simulink library "Library_SII_2018"  (R2018b)
settings: Solver=ode45  StartTime=0.0  StopTime=10.0  RelTol=1e-3  EnableMultiTasking=on
undefined symbols (not defined in the file or in its folder): coder, gcbh, r, simscape
libraries: fl_lib x157, nesl_utility x81, Library_SII2 x44, simulink x17, powerlib x12, mblibv1 x11, Simscape_SII_lib x11, elec_lib x10, Pneumatic_lib x4, $bdroot x2, peRmsMeasurement x1, powerlib_extras x1
(part 5 of 6)

== system Library_SII_2018/Mécanique/Engrenage droit SS ==
  Capteur de puissance mécanique de rotation : Subsystem  mask(Capteur de puissance mécanique de rotation){}
      mask help:
      | Le bloc représente un capteur de puissance mécanique de rotation.
      | R et C sont des ports physiques conservatifs.
      |
      | P, T et W sont des ports Simulink délivrant les valeurs de :
      |  - la puissance mécanique traversant le bloc (en W)
      |  - le couple transmis à travers le bloc (en Nm)
      |  - la vitesse de rotation (en rad/s)
      |
      | Ces valeurs sont calculées par rapport au référentiel Ref.
      mask Display:
      | plot([149.600878633536;150.016472378793;150.47508104106;150.972287968219;151.50330478576;152.063017511447;152.646035805762;153.246744883819;153.859359588817;154.477980106257;155.096648782383;155.709407499646;156.310355056631;156.893703999851;157.453836360095;157.985357756531;158.483149347555;158.942417128023;159.358738098149;159.728102859405;160.046954227227;160.312221488639;160.521349974904;160.672325664379;160.763694578642;160.794576785101;160.764674871227;160.674276808796;160.524253180566;160.316048796087;160.051668777399;159.733659248606;159.365082815313;158.949489070056;158.490880407788;157.993673480629;157.462656663088;156.908284800231], [156.971389291536;157.430657072004;157.84697804213;158.216342803387;158.535194171208;158.80046143262;159.009589918885;159.16056560836;159.251934522623;159.282816729083;159.252914815208;159.162516752777;159.012493124547;158.804288740068;158.53990872138;158.221899192587;157.853322759294;157.437729014037;156.979120351769;156.48191342461;155.950896607069;155.391183881382;154.808165587067;154.20745650901;153.594841804012;152.976221286573;152.357552610446;151.744793893183;151.143846336199;150.560497392978;150.000365032735;149.468843636298;148.971052045274;148.511784264806;148.095463294681;147.726098533424;147.407247165603;147.144199990631])
      | plot([152.057635404444;152.93604260309;153.834625296826;154.744729643097;155.657590839533;156.564417533794;157.45647648909;158.325176690034;159.162152078811;159.959342124889;160.709069452336;161.404113777147;162.037781442523;162.603969882449;163.097226392739;163.512800643557;163.846690427691;164.095680203997;164.257372064819;164.330208829146;164.313489039122;164.27939575172], [142.228020686971;141.979030910664;141.817339049842;141.744502285515;141.761222075539;141.867337399197;142.061826307913;142.342815767178;142.707599694895;143.152665022428;143.673725527376;144.265763112236;144.923076131425;145.639334301243;146.40763966397;147.220593018964;148.070365181011;148.948772379657;149.847355073393;150.757459419663;151.6703206161;152.055850472277])
      | %plot([116.468514315784;116.438789536125;116.349901463023;116.202706137216;115.998621130155;115.739611892022;115.42817282337;115.067303252679;114.660478551187;114.211616663162;113.725040373958;113.205435679231;112.657806656235;112.087427271827;111.499790591278;110.900555877058;110.29549408704;109.690432297022;109.091197582803;108.503560902254;107.933181517846;107.38555249485;106.865947800123;106.379371510919;105.930509622894;105.523684921402;105.162815350711;104.851376282059;104.592367043926;104.388282036865;104.241086711057;104.152198637956;104.122473858297;104.152198637956;104.241086711057;104.388282036865;104.592367043926;104.851376282059;105.162815350711;105.523684921402;105.930509622894;106.379371510919;106.865947800123;107.38555249485;107.933181517846;108.503560902254;109.091197582803;109.690432297022;110.29549408704;110.900555877058;111.499790591278;112.087427271827;112.657806656235;113.205435679231;113.725040373958;114.211616663162;114.660478551187;115.067303252679;115.42817282337;115.739611892022;115.998621130155;116.202706137216;116.349901463023;116.438789536125;116.468514315784;116.468514315784], [111.618284136057;111.013222346039;110.413987631819;109.826350951271;109.255971566862;108.708342543866;108.188737849139;107.702161559936;107.253299671911;106.846474970419;106.485605399728;106.174166331075;105.915157092943;105.711072085881;105.563876760074;105.474988686973;105.445263907313;105.474988686973;105.563876760074;105.711072085881;105.915157092943;106.174166331075;106.485605399728;106.846474970419;107.253299671911;107.702161559936;108.188737849139;108.708342543866;109.255971566862;109.826350951271;110.413987631819;111.013222346039;111.618284136057;112.223345926075;112.822580640295;113.410217320843;113.980596705252;114.528225728247;115.047830422975;115.534406712178;115.983268600203;116.390093301695;116.750962872386;117.062401941038;117.321411179171;117.525496186232;117.67269151204;117.761579585141;117.7913043648;117.761579585141;117.67269151204;117.525496186232;117.321411179171;117.062401941038;116.750962872386;116.390093301695;115.983268600203;115.534406712178;115.047830422975;114.528225728247;113.980596705252;113.410217320843;112.822580640295;112.223345926075;111.618284136057;111.618284136057])
      | plot([239.23602886498;238.828071429858;237.608127977604;235.587947230552;232.78698463364;229.232214987837;224.957872668068;220.005121927465;214.421660463109;208.261260061133;201.583248745024;194.451939414329;186.936010476274;179.107844435155;171.042830809261;162.818640088593;154.514475725591;146.210311362589;137.986120641921;129.921107016027;122.092940974909;114.577012036853;107.445702706158;100.76769139005;94.607290988073;89.0238295237172;84.0710787831142;79.7967364633452;76.2419668175427;73.4410042206305;71.4208234735788;70.2008800213248;69.7929225862026;70.2008800213248;71.4208234735788;73.4410042206306;76.2419668175428;79.7967364633454;84.0710787831144;89.0238295237174;94.6072909880733;100.76769139005;107.445702706159;114.577012036853;122.092940974909;129.921107016027;137.986120641921;146.210311362589;154.514475725591;162.818640088593;171.042830809261;179.107844435155;186.936010476274;194.451939414329;201.583248745024;208.261260061133;214.421660463109;220.005121927465;224.957872668068;229.232214987837;232.78698463364;235.587947230552;237.608127977604;238.828071429858;239.23602886498;239.23602886498], [155.774275772274;147.47628550917;139.258209428443;131.199192095207;123.376846251889;115.866505365088;108.740498123116;102.067451871182;95.9116316925529;90.3323215006612;85.3832531026163;81.1120887325275;77.5599620381344;74.7610819412943;72.742403187363;71.5233667562631;71.1157126352191;71.5233667562631;72.742403187363;74.7610819412943;77.5599620381345;81.1120887325275;85.3832531026164;90.3323215006612;95.9116316925529;102.067451871182;108.740498123116;115.866505365089;123.376846251889;131.199192095207;139.258209428443;147.47628550917;155.774275772274;164.072266035377;172.290342116104;180.34935944934;188.171705292658;195.682046179459;202.808053421432;209.481099673365;215.636919851994;221.216230043886;226.165298441931;230.43646281202;233.988589506413;236.787469603253;238.806148357184;240.025184788284;240.432838909328;240.025184788284;238.806148357184;236.787469603253;233.988589506413;230.43646281202;226.165298441931;221.216230043886;215.636919851994;209.481099673365;202.808053421432;195.682046179459;188.171705292658;180.34935944934;172.290342116105;164.072266035378;155.774275772274;155.774275772274])
      | plot([252.715889364481;252.243022716633;250.828976737403;248.487369462568;245.240751850236;241.120390602797;236.165967051481;230.425195003451;223.953361231755;216.812793033479;209.072257983804;200.806301666664;192.094529760025;183.020841389688;173.672621134841;164.139897466795;154.514475725591;144.889053984387;135.356330316341;126.008110061494;116.934421691157;108.222649784518;99.9566934673787;92.2161584177032;85.075590219427;78.6037564477313;72.8629843997015;67.9085608483856;63.7881996009461;60.5415819886144;58.199974713779;56.7859287345493;56.3130620867014;56.7859287345493;58.1999747137791;60.5415819886146;63.7881996009463;67.9085608483858;72.8629843997018;78.6037564477315;85.0755902194273;92.2161584177035;99.9566934673791;108.222649784519;116.934421691157;126.008110061494;135.356330316341;144.889053984387;154.514475725591;164.139897466796;173.672621134841;183.020841389688;192.094529760025;200.806301666664;209.072257983803;216.812793033479;223.953361231755;230.425195003451;236.165967051481;241.120390602797;245.240751850236;248.487369462568;250.828976737403;252.243022716633;252.715889364481;252.715889364481], [154.514475725591;144.895228084285;135.36861905618;126.026395093992;116.958526921455;108.252343066071;99.9916888376535;92.2561188521535;85.1201308772245;78.6524483779929;72.9153586725213;67.9641130708855;63.8463947748555;60.6018596625959;58.2617543808809;56.8486154228053;56.3760520890355;56.8486154228053;58.2617543808809;60.6018596625959;63.8463947748555;67.9641130708856;72.9153586725213;78.652448377993;85.1201308772246;92.2561188521536;99.9916888376536;108.252343066072;116.958526921455;126.026395093992;135.36861905618;144.895228084285;154.514475725591;164.133723366898;173.660332395002;183.002556357191;192.070424529728;200.776608385111;209.037262613529;216.772832599029;223.908820573958;230.37650307319;236.113592778661;241.064838380297;245.182556676327;248.427091788587;250.767197070302;252.180336028377;252.652899362147;252.180336028377;250.767197070301;248.427091788587;245.182556676327;241.064838380297;236.113592778661;230.37650307319;223.908820573958;216.772832599029;209.037262613529;200.776608385111;192.070424529728;183.002556357191;173.660332395002;164.133723366898;154.514475725592;154.514475725591])
      | plot([154.514475725591;129.948374815285;179.017586633563;154.514475725591], [240.369848906994;203.583687543869;203.583687543869;240.369848906994])
      | %plot([105.382273904979;149.60125554353], [115.271704271436;156.971085816622])
      | plot([144.688035361469;144.688035361469], [152.057865634561;203.583687543869])
      | plot([164.277926087379;164.277926087379], [152.057865634561;203.583687543869])
      | plot([159.112745895982;159.616665914655], [149.60125554353;149.60125554353])
      | %plot([115.208714269102;159.364705905318], [107.901873998344;149.60125554353])
      | plot([0;311.800511553884;311.800511553884;0;0], [311.800511553884;311.800511553884;0;0;311.800511553884])
      | ;
      | color('red');
      | port_label('LConn', 1,'R')
      | port_label('RConn', 1,'C')
      | port_label('LConn', 2,'Ref')
      | port_label('output', 1,'P')
      | port_label('output', 2,'T')
      | port_label('output', 3,'W')
      | %port_label('RConn', 3,'A')
  Couple d'entrée : Scope
  Couple de sortie : Scope
  Gain : Gain  Gain=1-n
  Gear Box : fl_lib/Mechanical/Mechanisms/Gear Box  ratio=r  t_in_specify=off  t_in_priority=High  t_in=0 N*m  t_in_nominal_specify=off  t_in_nominal_unit=N*m  t_in_nominal_value=1  t_out_specify=off  t_out_priority=High  t_out=0 N*m  t_out_nominal_specify=off  t_out_nominal_unit=N*m  t_out_nominal_value=1
  Ideal Torque Source : fl_lib/Mechanical/Mechanical Sources/Ideal Torque Source
  Inertia : fl_lib/Mechanical/Rotational Elements/Inertia  inertia=J kg*m^2  w_specify=on  w_priority=High  w=0 rad/s  w_nominal_specify=off  w_nominal_unit=rad/s  w_nominal_value=1  t_specify=off  t_priority=High  t=0 N*m  t_nominal_specify=off  t_nominal_unit=N*m  t_nominal_value=1
  Simulink-PS Converter : nesl_utility/Simulink-PS Converter  PhysicalDomain=network_engine_domain  SubClassName=ps_input  LeftPortType=input  RightPortType=output  PseudoPeriodic=off  Frequencies=[]  NoiseDistribution=none  NoiseParameters=[]  Unit=1  AffineConversion=off  FilteringAndDerivatives=zero  SimscapeFilterOrder=1  InputFilterTimeConstant=.001  UdotUserProvided=0
  R : PMIOPort  Side=Right
  V : PMIOPort  Tag=PMCPort  Port=2  Side=Left
  Ref : PMIOPort  Tag=PMCPort  Port=3  Side=Left
  wires:
  Capteur de puissance mécanique de rotation/2(C) -> Gain/1, Couple d'entrée/1
  Gain/1 -> Simulink-PS Converter/1, Couple de sortie/1
  connections:
  V/RConn1 -- Capteur de puissance mécanique de rotation/LConn2
  Capteur de puissance mécanique de rotation/LConn1 -- Ideal Torque Source/RConn2 -- Ref/RConn1
  R/RConn1 -- Gear Box/RConn1
  Simulink-PS Converter/RConn1 -- Ideal Torque Source/RConn1
  Inertia/LConn1 -- Gear Box/LConn1 -- Ideal Torque Source/LConn1 -- Capteur de puissance mécanique de rotation/RConn1

== system Library_SII_2018/Mécanique/Roue - Vis sans fin SS ==
  Capteur de puissance mécanique de rotation : Subsystem  mask(Capteur de puissance mécanique de rotation){}
      mask help:
      | Le bloc représente un capteur de puissance mécanique de rotation.
      | R et C sont des ports physiques conservatifs.
      |
      | P, T et W sont des ports Simulink délivrant les valeurs de :
      |  - la puissance mécanique traversant le bloc (en W)
      |  - le couple transmis à travers le bloc (en Nm)
      |  - la vitesse de rotation (en rad/s)
      |
      | Ces valeurs sont calculées par rapport au référentiel Ref.
      mask Display:
      | plot([149.600878633536;150.016472378793;150.47508104106;150.972287968219;151.50330478576;152.063017511447;152.646035805762;153.246744883819;153.859359588817;154.477980106257;155.096648782383;155.709407499646;156.310355056631;156.893703999851;157.453836360095;157.985357756531;158.483149347555;158.942417128023;159.358738098149;159.728102859405;160.046954227227;160.312221488639;160.521349974904;160.672325664379;160.763694578642;160.794576785101;160.764674871227;160.674276808796;160.524253180566;160.316048796087;160.051668777399;159.733659248606;159.365082815313;158.949489070056;158.490880407788;157.993673480629;157.462656663088;156.908284800231], [156.971389291536;157.430657072004;157.84697804213;158.216342803387;158.535194171208;158.80046143262;159.009589918885;159.16056560836;159.251934522623;159.282816729083;159.252914815208;159.162516752777;159.012493124547;158.804288740068;158.53990872138;158.221899192587;157.853322759294;157.437729014037;156.979120351769;156.48191342461;155.950896607069;155.391183881382;154.808165587067;154.20745650901;153.594841804012;152.976221286573;152.357552610446;151.744793893183;151.143846336199;150.560497392978;150.000365032735;149.468843636298;148.971052045274;148.511784264806;148.095463294681;147.726098533424;147.407247165603;147.144199990631])
      | plot([152.057635404444;152.93604260309;153.834625296826;154.744729643097;155.657590839533;156.564417533794;157.45647648909;158.325176690034;159.162152078811;159.959342124889;160.709069452336;161.404113777147;162.037781442523;162.603969882449;163.097226392739;163.512800643557;163.846690427691;164.095680203997;164.257372064819;164.330208829146;164.313489039122;164.27939575172], [142.228020686971;141.979030910664;141.817339049842;141.744502285515;141.761222075539;141.867337399197;142.061826307913;142.342815767178;142.707599694895;143.152665022428;143.673725527376;144.265763112236;144.923076131425;145.639334301243;146.40763966397;147.220593018964;148.070365181011;148.948772379657;149.847355073393;150.757459419663;151.6703206161;152.055850472277])
      | %plot([116.468514315784;116.438789536125;116.349901463023;116.202706137216;115.998621130155;115.739611892022;115.42817282337;115.067303252679;114.660478551187;114.211616663162;113.725040373958;113.205435679231;112.657806656235;112.087427271827;111.499790591278;110.900555877058;110.29549408704;109.690432297022;109.091197582803;108.503560902254;107.933181517846;107.38555249485;106.865947800123;106.379371510919;105.930509622894;105.523684921402;105.162815350711;104.851376282059;104.592367043926;104.388282036865;104.241086711057;104.152198637956;104.122473858297;104.152198637956;104.241086711057;104.388282036865;104.592367043926;104.851376282059;105.162815350711;105.523684921402;105.930509622894;106.379371510919;106.865947800123;107.38555249485;107.933181517846;108.503560902254;109.091197582803;109.690432297022;110.29549408704;110.900555877058;111.499790591278;112.087427271827;112.657806656235;113.205435679231;113.725040373958;114.211616663162;114.660478551187;115.067303252679;115.42817282337;115.739611892022;115.998621130155;116.202706137216;116.349901463023;116.438789536125;116.468514315784;116.468514315784], [111.618284136057;111.013222346039;110.413987631819;109.826350951271;109.255971566862;108.708342543866;108.188737849139;107.702161559936;107.253299671911;106.846474970419;106.485605399728;106.174166331075;105.915157092943;105.711072085881;105.563876760074;105.474988686973;105.445263907313;105.474988686973;105.563876760074;105.711072085881;105.915157092943;106.174166331075;106.485605399728;106.846474970419;107.253299671911;107.702161559936;108.188737849139;108.708342543866;109.255971566862;109.826350951271;110.413987631819;111.013222346039;111.618284136057;112.223345926075;112.822580640295;113.410217320843;113.980596705252;114.528225728247;115.047830422975;115.534406712178;115.983268600203;116.390093301695;116.750962872386;117.062401941038;117.321411179171;117.525496186232;117.67269151204;117.761579585141;117.7913043648;117.761579585141;117.67269151204;117.525496186232;117.321411179171;117.062401941038;116.750962872386;116.390093301695;115.983268600203;115.534406712178;115.047830422975;114.528225728247;113.980596705252;113.410217320843;112.822580640295;112.223345926075;111.618284136057;111.618284136057])
      | plot([239.23602886498;238.828071429858;237.608127977604;235.587947230552;232.78698463364;229.232214987837;224.957872668068;220.005121927465;214.421660463109;208.261260061133;201.583248745024;194.451939414329;186.936010476274;179.107844435155;171.042830809261;162.818640088593;154.514475725591;146.210311362589;137.986120641921;129.921107016027;122.092940974909;114.577012036853;107.445702706158;100.76769139005;94.607290988073;89.0238295237172;84.0710787831142;79.7967364633452;76.2419668175427;73.4410042206305;71.4208234735788;70.2008800213248;69.7929225862026;70.2008800213248;71.4208234735788;73.4410042206306;76.2419668175428;79.7967364633454;84.0710787831144;89.0238295237174;94.6072909880733;100.76769139005;107.445702706159;114.577012036853;122.092940974909;129.921107016027;137.986120641921;146.210311362589;154.514475725591;162.818640088593;171.042830809261;179.107844435155;186.936010476274;194.451939414329;201.583248745024;208.261260061133;214.421660463109;220.005121927465;224.957872668068;229.232214987837;232.78698463364;235.587947230552;237.608127977604;238.828071429858;239.23602886498;239.23602886498], [155.774275772274;147.47628550917;139.258209428443;131.199192095207;123.376846251889;115.866505365088;108.740498123116;102.067451871182;95.9116316925529;90.3323215006612;85.3832531026163;81.1120887325275;77.5599620381344;74.7610819412943;72.742403187363;71.5233667562631;71.1157126352191;71.5233667562631;72.742403187363;74.7610819412943;77.5599620381345;81.1120887325275;85.3832531026164;90.3323215006612;95.9116316925529;102.067451871182;108.740498123116;115.866505365089;123.376846251889;131.199192095207;139.258209428443;147.47628550917;155.774275772274;164.072266035377;172.290342116104;180.34935944934;188.171705292658;195.682046179459;202.808053421432;209.481099673365;215.636919851994;221.216230043886;226.165298441931;230.43646281202;233.988589506413;236.787469603253;238.806148357184;240.025184788284;240.432838909328;240.025184788284;238.806148357184;236.787469603253;233.988589506413;230.43646281202;226.165298441931;221.216230043886;215.636919851994;209.481099673365;202.808053421432;195.682046179459;188.171705292658;180.34935944934;172.290342116105;164.072266035378;155.774275772274;155.774275772274])
      | plot([252.715889364481;252.243022716633;250.828976737403;248.487369462568;245.240751850236;241.120390602797;236.165967051481;230.425195003451;223.953361231755;216.812793033479;209.072257983804;200.806301666664;192.094529760025;183.020841389688;173.672621134841;164.139897466795;154.514475725591;144.889053984387;135.356330316341;126.008110061494;116.934421691157;108.222649784518;99.9566934673787;92.2161584177032;85.075590219427;78.6037564477313;72.8629843997015;67.9085608483856;63.7881996009461;60.5415819886144;58.199974713779;56.7859287345493;56.3130620867014;56.7859287345493;58.1999747137791;60.5415819886146;63.7881996009463;67.9085608483858;72.8629843997018;78.6037564477315;85.0755902194273;92.2161584177035;99.9566934673791;108.222649784519;116.934421691157;126.008110061494;135.356330316341;144.889053984387;154.514475725591;164.139897466796;173.672621134841;183.020841389688;192.094529760025;200.806301666664;209.072257983803;216.812793033479;223.953361231755;230.425195003451;236.165967051481;241.120390602797;245.240751850236;248.487369462568;250.828976737403;252.243022716633;252.715889364481;252.715889364481], [154.514475725591;144.895228084285;135.36861905618;126.026395093992;116.958526921455;108.252343066071;99.9916888376535;92.2561188521535;85.1201308772245;78.6524483779929;72.9153586725213;67.9641130708855;63.8463947748555;60.6018596625959;58.2617543808809;56.8486154228053;56.3760520890355;56.8486154228053;58.2617543808809;60.6018596625959;63.8463947748555;67.9641130708856;72.9153586725213;78.652448377993;85.1201308772246;92.2561188521536;99.9916888376536;108.252343066072;116.958526921455;126.026395093992;135.36861905618;144.895228084285;154.514475725591;164.133723366898;173.660332395002;183.002556357191;192.070424529728;200.776608385111;209.037262613529;216.772832599029;223.908820573958;230.37650307319;236.113592778661;241.064838380297;245.182556676327;248.427091788587;250.767197070302;252.180336028377;252.652899362147;252.180336028377;250.767197070301;248.427091788587;245.182556676327;241.064838380297;236.113592778661;230.37650307319;223.908820573958;216.772832599029;209.037262613529;200.776608385111;192.070424529728;183.002556357191;173.660332395002;164.133723366898;154.514475725592;154.514475725591])
      | plot([154.514475725591;129.948374815285;179.017586633563;154.514475725591], [240.369848906994;203.583687543869;203.583687543869;240.369848906994])
      | %plot([105.382273904979;149.60125554353], [115.271704271436;156.971085816622])
      | plot([144.688035361469;144.688035361469], [152.057865634561;203.583687543869])
      | plot([164.277926087379;164.277926087379], [152.057865634561;203.583687543869])
      | plot([159.112745895982;159.616665914655], [149.60125554353;149.60125554353])
      | %plot([115.208714269102;159.364705905318], [107.901873998344;149.60125554353])
      | plot([0;311.800511553884;311.800511553884;0;0], [311.800511553884;311.800511553884;0;0;311.800511553884])
      | ;
      | color('red');
      | port_label('LConn', 1,'R')
      | port_label('RConn', 1,'C')
      | port_label('LConn', 2,'Ref')
      | port_label('output', 1,'P')
      | port_label('output', 2,'T')
      | port_label('output', 3,'W')
      | %port_label('RConn', 3,'A')
  Fcn : Fcn  Expr=0.5*((u-1)*(1-n2)+(u+1)*(1-n1))
  Gear Box : fl_lib/Mechanical/Mechanisms/Gear Box  ratio=r  t_in_specify=off  t_in_priority=High  t_in=0 N*m  t_in_nominal_specify=off  t_in_nominal_unit=N*m  t_in_nominal_value=1  t_out_specify=off  t_out_priority=High  t_out=0 N*m  t_out_nominal_specify=off  t_out_nominal_unit=N*m  t_out_nominal_value=1
  Ideal Rotational Motion Sensor : fl_lib/Mechanical/Mechanical Sensors/Ideal Rotational Motion Sensor  offset=0 rad
  Ideal Torque Source : fl_lib/Mechanical/Mechanical Sources/Ideal Torque Source
  Inertia : fl_lib/Mechanical/Rotational Elements/Inertia  inertia=J kg*m^2  w_specify=on  w_priority=High  w=0 rad/s  w_nominal_specify=off  w_nominal_unit=rad/s  w_nominal_value=1  t_specify=off  t_priority=High  t=0 N*m  t_nominal_specify=off  t_nominal_unit=N*m  t_nominal_value=1
  Product : Product  RndMeth=Zero
  Scope : Scope
  Scope1 : Scope
  Sign : Signum
  Simulink-PS Converter : nesl_utility/Simulink-PS Converter  PhysicalDomain=network_engine_domain  SubClassName=ps_input  LeftPortType=input  RightPortType=output  PseudoPeriodic=off  Frequencies=[]  NoiseDistribution=none  NoiseParameters=[]  Unit=1  AffineConversion=off  FilteringAndDerivatives=zero  SimscapeFilterOrder=1  InputFilterTimeConstant=.001  UdotUserProvided=0
  R : PMIOPort  Side=Right
  V : PMIOPort  Tag=PMCPort  Port=2  Side=Left
  Ref : PMIOPort  Tag=PMCPort  Port=3  Side=Left
  wires:
  Capteur de puissance mécanique de rotation/2(C) -> Scope1/1, Product/2
  Fcn/1 -> Product/1
  Product/1 -> Simulink-PS Converter/1, Scope/1
  Sign/1 -> Fcn/1
  Capteur de puissance mécanique de rotation/1(P) -> Sign/1
  connections:
  V/RConn1 -- Capteur de puissance mécanique de rotation/LConn2
  Capteur de puissance mécanique de rotation/LConn1 -- Ideal Torque Source/RConn2 -- Ref/RConn1
  R/RConn1 -- Gear Box/RConn1
  Simulink-PS Converter/RConn1 -- Ideal Torque Source/RConn1
  Gear Box/LConn1 -- Ideal Torque Source/LConn1 -- Capteur de puissance mécanique de rotation/RConn1 -- Inertia/LConn1

== system Library_SII_2018/Mécanique/Roue libre SM ==
  Add1 : Sum
  Constant : Constant  Value=0
  Constant1 : Constant  Value=0
  Constant2 : Constant  Value=inf
  Constante de frottement : Constant  Value=kv
  "Couple constant pour maintenir la roue libre en position \"bloquee\" en l'absence de couple transmis" : Constant  Value=1e-10
  Gain1 : Gain  Gain=-1  SaturateOnIntegerOverflow=on  OutDataTypeStr=Inherit: Same as input  ParamDataTypeStr=Inherit: Same as input
  Joint Stiction Actuator : mblibv1/Sensors &  Actuators/Joint Stiction Actuator  UpdateFromCAD=off  PhysicalDomain=Mechanical  PortType=blob  ActuationStyle=Force  AngleUnits=deg  ArcVelocityUnits=deg/s  ArcAccelerationUnits=deg/s^2  CoordPositionUnits=m  VelocityUnits=m/s  AccelerationUnits=m/s^2  ForceUnits=N  TorqueUnits=N-m  ActiveIO=off  Width=5  DialogClass=EventActuatorBlock  Primitive=R1  FrictionalForceUnits=N  ExternalForceUnits=N  FrictionalTorqueUnits=N*m  ExternalTorqueUnits=N*m  LockingTolerance=1e-2
      settings: SourceProductName=Simscape Multibody  SourceProductBaseCode=MS
  Mesures : mblibv1/Sensors &  Actuators/Joint Sensor  UpdateFromCAD=off  PhysicalDomain=Mechanical  PortType=blob  Muxed=off  Pose=off  Angle=off  AngleUnits=deg  ArcVelocity=on  ArcVelocityUnits=rad/s  ArcAcceleration=off  ArcAccelerationUnits=deg/s^2  CoordPosition=on  CoordPositionUnits=m  Velocity=off  VelocityUnits=m/s  Acceleration=off  AccelerationUnits=m/s^2  Quaternion=on  QuaternionDT=off  QuaternionDDT=off  QuaternionUnits=off  OutputVector=[1]  ActiveIO=off  Width=5  DialogClass=MechanicalSensorBlock  Primitive=R1  Force=off  ForceUnits=N  Torque=on  TorqueUnits=N*m  ReferenceFrame=Absolute (World)  ReactionSensedSide=Base  ReactionReferenceFrame=Absolute (World)  ReactionForce=off  ReactionForceUnits=N  ReactionMoment=off  ReactionMomentUnits=N*m
      settings: SourceProductName=Simscape Multibody  SourceProductBaseCode=MS
  Product2 : Product  SaturateOnIntegerOverflow=on  InputSameDT=on  OutDataTypeStr=Inherit: Same as first input
  Revolute : mblibv1/Joints/Revolute  LConnTagsString=__newl0|SA1  RConnTagsString=__newr0|SA1  UpdateFromCAD=off  NumSAPorts=2  CutJoint=off  MarkAsCut=off  Primitives=prismatic  PrimitiveProps=R1$World$axe$revolute  DialogClass=JointBlock  R1Axis=axe
      settings: SourceProductName=Simscape Multibody  SourceProductBaseCode=MS
  Scope : Scope
  F : PMIOPort  Side=Right
  B : PMIOPort  Port=2  Side=Left
  wires:
  Constant1/1 -> Joint Stiction Actuator/3
  "Couple constant pour maintenir la roue libre en position \"bloquee\" en l'absence de couple transmis"/1 -> Add1/2
  Product2/1 -> Joint Stiction Actuator/2
  Mesures/1 -> Gain1/1
  Mesures/2 -> Add1/1, Scope/1  "Couple transmis"
  Gain1/1 -> Product2/2
  Constante de frottement/1 -> Product2/1
  Add1/1 -> Joint Stiction Actuator/4
  Constant2/1 -> Joint Stiction Actuator/5
  Constant/1 -> Joint Stiction Actuator/1
  connections:
  Mesures/LConn1 -- Revolute/LConn2
  Revolute/RConn2 -- Joint Stiction Actuator/RConn1
  F/RConn1 -- Revolute/RConn1
  B/RConn1 -- Revolute/LConn1

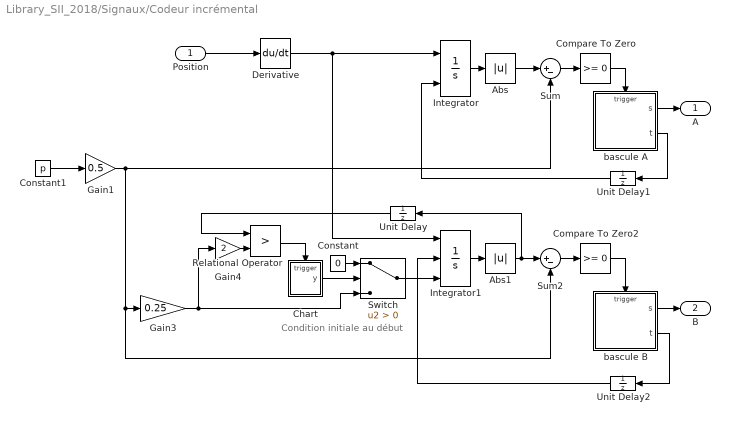
== system Library_SII_2018/Signaux/Codeur incrémental ==
  note: Condition initiale
      | au début
  Position : Inport
  Abs : Abs
  Abs1 : Abs
  Chart : Stateflow chart  TreatAsAtomicUnit=on
  Compare To Zero : simulink/Logic and Bit Operations/Compare To Zero  relop=>=  OutDataTypeStr=boolean
  Compare To Zero2 : simulink/Logic and Bit Operations/Compare To Zero  relop=>=  OutDataTypeStr=boolean
  Constant : Constant  Value=0
  Constant1 : Constant  Value=p
  Derivative : Derivative
  Gain1 : Gain  Gain=0.5
  Gain3 : Gain  Gain=0.25
  Gain4 : Gain  Gain=2
  Integrator : Integrator  ExternalReset=either
  Integrator1 : Integrator  ExternalReset=either  InitialConditionSource=external
  Relational Operator : RelationalOperator  Operator=>  OutDataTypeStr=boolean  RndMeth=Nearest
  Sum : Sum  Inputs=|+-
  Sum2 : Sum  Inputs=|+-
  Switch : Switch  Criteria=u2 > Threshold
  Unit Delay : UnitDelay  SampleTime=-1
  Unit Delay1 : UnitDelay  SampleTime=-1
  Unit Delay2 : UnitDelay  SampleTime=-1
  bascule A : Stateflow chart  TreatAsAtomicUnit=on
  bascule B : Stateflow chart  TreatAsAtomicUnit=on
  A : Outport
  B : Outport  Port=2
  wires:
  Unit Delay2/1 -> Integrator1/2
  bascule B/2(t) -> Unit Delay2/1
  Unit Delay1/1 -> Integrator/2
  Compare To Zero2/1 -> bascule B/Trigger
  bascule A/2(t) -> Unit Delay1/1
  Compare To Zero/1 -> bascule A/Trigger
  Gain1/1 -> Sum2/2, Gain3/1, Sum/2
  Position/1 -> Derivative/1
  Constant1/1 -> Gain1/1
  Gain4/1 -> Relational Operator/2
  Switch/1 -> Integrator1/3
  Constant/1 -> Switch/1
  Chart/1(y) -> Switch/2
  Unit Delay/1 -> Relational Operator/1
  Derivative/1 -> Integrator/1, Integrator1/1
  Relational Operator/1 -> Chart/Trigger
  Abs1/1 -> Sum2/1, Unit Delay/1
  Gain3/1 -> Switch/3, Gain4/1
  bascule B/1(s) -> B/1
  Integrator1/1 -> Abs1/1
  Sum2/1 -> Compare To Zero2/1
  bascule A/1(s) -> A/1
  Abs/1 -> Sum/1
  Integrator/1 -> Abs/1
  Sum/1 -> Compare To Zero/1

== system Library_SII_2018/Signaux/Contrôle de régime ==
  x : Inport
  Clock : Clock
  Constant : Constant  Value=al
  Constant1 : Constant  Value=vl
  Derivative : Derivative
  MATLAB Function : MATLAB Function  TreatAsAtomicUnit=on
  Memory : Memory
  Memory2 : Memory
  Memory5 : Memory
  Transfer Fcn4 : TransferFcn  Denominator=[1/(al*100)^2 2/(al*100) 1]
  xc : Outport
  wires:
  Clock/1 -> Memory5/1, MATLAB Function/1(t)
  Constant/1 -> MATLAB Function/4(al)
  Constant1/1 -> MATLAB Function/5(vl)
  x/1 -> MATLAB Function/3(x)
  Memory5/1 -> MATLAB Function/2(t_1)
  Memory/1 -> MATLAB Function/6(x_1)
  Derivative/1 -> Memory2/1
  MATLAB Function/1(xc) -> Transfer Fcn4/1, Memory/1, Derivative/1
  Memory2/1 -> MATLAB Function/7(v_1)
  Transfer Fcn4/1 -> xc/1

== system Library_SII_2018/Signaux/Frequence-Metre ==
  Signal : Inport
  Constant : Constant  Value=1/Ts
  Constant1 : Constant  Value=spec
  Constant2 : Constant  Value=plage
  Discrete Shift Register : powerlib_extras/Discrete  Control Blocks/Discrete Shift Register  NSamples=N  InitialValue=0  Ts=Ts
  MATLAB Function : MATLAB Function  TreatAsAtomicUnit=on
  Reshape : Reshape  OutputDimensionality=Customize  OutputDimensions=[1,N]
  TsFFT1 : ZeroOrderHold
  Frequence : Outport
  Amplitude : Outport  Port=2
  wires:
  Constant1/1 -> MATLAB Function/3(spec)
  Constant2/1 -> MATLAB Function/4(plage)
  Constant/1 -> MATLAB Function/2(fs)
  MATLAB Function/2(Pmax) -> Amplitude/1
  MATLAB Function/1(F) -> Frequence/1
  Signal/1 -> Discrete Shift Register/1
  TsFFT1/1 -> MATLAB Function/1(x)
  Reshape/1 -> TsFFT1/1
  Discrete Shift Register/1 -> Reshape/1

== system Library_SII_2018/Signaux/Générateur de signal carré ==
  Add1 : Sum
  Step : Step  Time=t  After=a  SampleTime=0
  Step1 : Step  Time=d+t  After=-a  SampleTime=0
  Out1 : Outport
  wires:
  Add1/1 -> Out1/1
  Step1/1 -> Add1/2
  Step/1 -> Add1/1

== system Library_SII_2018/Signaux/Générateur de signal pas ==
  Add1 : Sum
  Ramp : simulink/Sources/Ramp  slope=-p  start=a/p  InitialOutput=0
  Ramp1 : simulink/Sources/Ramp  slope=p  start=t  InitialOutput=0
  Out1 : Outport
  wires:
  Add1/1 -> Out1/1
  Ramp/1 -> Add1/2
  Ramp1/1 -> Add1/1

== system Library_SII_2018/Signaux/Générateur de signal périodique carré ==
  Fréquence [Hz] : Inport
  Rapport cyclique (0-1) : Inport  Port=2
  Compare To Zero : simulink/Logic and Bit Operations/Compare To Zero  relop=>=  OutDataTypeStr=boolean
  Constant : Constant
  Constant1 : Constant
  Gain : Gain  Gain=0.5
  Integrator : Integrator  ExternalReset=rising
  Sign : Signum
  Sum : Sum  Inputs=|+-
  Sum1 : Sum  Inputs=|-+
  Sum2 : Sum  Inputs=|++
  S : Outport
  wires:
  Rapport cyclique (0-1)/1 -> Sum1/2
  Compare To Zero/1 -> Integrator/2
  Sum1/1 -> Sign/1
  Constant1/1 -> Sum2/2
  Integrator/1 -> Sum1/1, Sum/1
  Gain/1 -> S/1
  Sign/1 -> Sum2/1
  Sum2/1 -> Gain/1
  Fréquence [Hz]/1 -> Integrator/1
  Constant/1 -> Sum/2
  Sum/1 -> Compare To Zero/1

== system Library_SII_2018/Signaux/Signal carré périodique symétrique ==
  Add : Sum  Inputs=+-
  Constant : Constant  Value=a
  Pulse Generator : DiscretePulseGenerator  PulseType=Time based  Amplitude=2*a  Period=T  PulseWidth=r
  Out1 : Outport
  wires:
  Constant/1 -> Add/2
  Pulse Generator/1 -> Add/1
  Add/1 -> Out1/1

== system Library_SII_2018/Signaux/Trapèze ==
  Add : Sum  Inputs=++++
  Ramp : simulink/Sources/Ramp  slope=p  start=t0  InitialOutput=0
  Ramp1 : simulink/Sources/Ramp  slope=-p  start=t0+a/p  InitialOutput=0
  Ramp2 : simulink/Sources/Ramp  slope=-p  start=t0+th+a/p  InitialOutput=0
  Ramp3 : simulink/Sources/Ramp  slope=p  start=t0+th+2*a/p  InitialOutput=0
  Out1 : Outport
  wires:
  Ramp3/1 -> Add/4
  Ramp2/1 -> Add/3
  Add/1 -> Out1/1
  Ramp/1 -> Add/1
  Ramp1/1 -> Add/2

== system Library_SII_2018/ThermLiquid/Capteur Pression Température [bar] et [°C] ==
  Absolute Reference (TL) : fl_lib/Thermal Liquid/Elements/Absolute Reference (TL)
      settings: SourceProductName=Simscape  SourceProductBaseCode=SS
  Fcn : Fcn  Expr=u-273.16
  PS-Simulink Converter : nesl_utility/PS-Simulink Converter  PhysicalDomain=network_engine_domain  SubClassName=ps_output  LeftPortType=input  RightPortType=output  PseudoPeriodic=off  Frequencies=[]  Unit=bar  AffineConversion=off
  PS-Simulink Converter1 : nesl_utility/PS-Simulink Converter  PhysicalDomain=network_engine_domain  SubClassName=ps_output  LeftPortType=input  RightPortType=output  PseudoPeriodic=off  Frequencies=[]  Unit=1  AffineConversion=off
  Pressure & Temperature Sensor (TL) : fl_lib/Thermal Liquid/Sensors/Pressure & Temperature Sensor (TL)
      settings: SourceProductName=Simscape  SourceProductBaseCode=SS
  S : PMIOPort  Side=Left
  p [bar] : Outport
  T [°C] : Outport  Port=2
  wires:
  PS-Simulink Converter1/1 -> Fcn/1
  PS-Simulink Converter/1 -> p [bar]/1
  Fcn/1 -> T [°C]/1
  connections:
  PS-Simulink Converter1/LConn1 -- Pressure & Temperature Sensor (TL)/RConn3
  PS-Simulink Converter/LConn1 -- Pressure & Temperature Sensor (TL)/RConn2
  Absolute Reference (TL)/LConn1 -- Pressure & Temperature Sensor (TL)/RConn1
  S/RConn1 -- Pressure & Temperature Sensor (TL)/LConn1

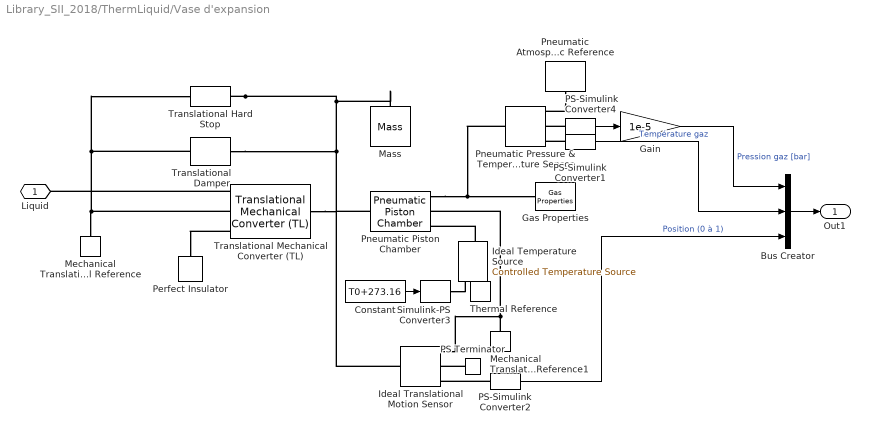
== system Library_SII_2018/ThermLiquid/Vase d'expansion ==
  Bus Creator : BusCreator  Inputs=3
  Constant : Constant  Value=T0+273.16
  Gain : Gain  Gain=1e-5
  Gas Properties : Pneumatic_lib/Pneumatic Utilities/Gas Properties  c_p=1005 J/kg/K  c_v=717.95 J/kg/K  viscosity=18.21e-6 s*Pa  Pa=1 atm  Ta=20 C  range_error=2
      settings: SourceProductName=Simscape  SourceProductBaseCode=SS
  Ideal Temperature Source : fl_lib/Thermal/Thermal Sources/Controlled Temperature Source
      settings: SourceProductName=Simscape
  Ideal Translational Motion Sensor : fl_lib/Mechanical/Mechanical Sensors/Ideal Translational Motion Sensor  offset=0 m
  Mass : fl_lib/Mechanical/Translational Elements/Mass  mass=0.05 kg  v_specify=off  v_priority=High  v=0 m/s  v_nominal_specify=off  v_nominal_unit=m/s  v_nominal_value=1  f_specify=off  f_priority=High  f=0 N  f_nominal_specify=off  f_nominal_unit=N  f_nominal_value=1
  Mechanical Translational Reference : fl_lib/Mechanical/Translational Elements/Mechanical Translational Reference
  Mechanical Translational Reference1 : fl_lib/Mechanical/Translational Elements/Mechanical Translational Reference
  PS Terminator : fl_lib/Physical Signals/Sinks/PS Terminator
      settings: SourceProductName=Simscape
  PS-Simulink Converter1 : nesl_utility/PS-Simulink Converter  PhysicalDomain=network_engine_domain  SubClassName=ps_output  LeftPortType=input  RightPortType=output  PseudoPeriodic=off  Frequencies=[]  Unit=1  AffineConversion=off
  PS-Simulink Converter2 : nesl_utility/PS-Simulink Converter  PhysicalDomain=network_engine_domain  SubClassName=ps_output  LeftPortType=input  RightPortType=output  PseudoPeriodic=off  Frequencies=[]  Unit=1  AffineConversion=off
  PS-Simulink Converter4 : nesl_utility/PS-Simulink Converter  PhysicalDomain=network_engine_domain  SubClassName=ps_output  LeftPortType=input  RightPortType=output  PseudoPeriodic=off  Frequencies=[]  Unit=1  AffineConversion=off
  Perfect Insulator : fl_lib/Thermal/Thermal Elements/Perfect Insulator  T_specify=on  T_priority=High  T=T0 C  T_nominal_specify=off  T_nominal_unit=K  T_nominal_value=1
      settings: SourceProductName=Simscape
  Pneumatic Atmospheric Reference : Pneumatic_lib/Pneumatic Elements/Pneumatic Atmospheric Reference
      settings: SourceProductName=Simscape  SourceProductBaseCode=SS
  Pneumatic Piston Chamber : Pneumatic_lib/Pneumatic Elements/Pneumatic Piston Chamber  Area=V/1000 m^2  x0=1 m  V0=1e-5 m^3  or=2  pressure_specify=on  pressure_priority=High  pressure=p0 bar  pressure_nominal_specify=off  pressure_nominal_unit=Pa  pressure_nominal_value=1  temperature_specify=on  temperature_priority=High  temperature=T0 C  temperature_nominal_specify=off  temperature_nominal_unit=K  temperature_nominal_value=1  gas_flow_specify=off  gas_flow_priority=High  gas_flow=0 kg/s  gas_flow_nominal_specify=off  gas_flow_nominal_unit=kg/s  gas_flow_nominal_value=1  heat_flow_specify=off  heat_flow_priority=High  heat_flow=0 J/s  heat_flow_nominal_specify=off  heat_flow_nominal_unit=J/s  heat_flow_nominal_value=1  heat_exch_flow_specify=off  heat_exch_flow_priority=High  heat_exch_flow=0 J/s  heat_exch_flow_nominal_specify=off  heat_exch_flow_nominal_unit=J/s  heat_exch_flow_nominal_value=1  velocity_specify=off  velocity_priority=High  velocity=0 m/s  velocity_nominal_specify=off  velocity_nominal_unit=m/s  velocity_nominal_value=1  force_specify=off  force_priority=High  force=0 N  force_nominal_specify=off  force_nominal_unit=N  force_nominal_value=1
      settings: SourceProductName=Simscape  SourceProductBaseCode=SS
  Pneumatic Pressure & Temperature Sensor : Pneumatic_lib/Pneumatic Sensors/Pneumatic Pressure & Temperature Sensor
      settings: SourceProductName=Simscape  SourceProductBaseCode=SS
  Simulink-PS Converter3 : nesl_utility/Simulink-PS Converter  PhysicalDomain=network_engine_domain  SubClassName=ps_input  LeftPortType=input  RightPortType=output  PseudoPeriodic=off  Frequencies=[]  NoiseDistribution=none  NoiseParameters=[]  Unit=1  AffineConversion=off  FilteringAndDerivatives=zero  SimscapeFilterOrder=1  InputFilterTimeConstant=.001  UdotUserProvided=1
  Thermal Reference : fl_lib/Thermal/Thermal Elements/Thermal Reference
  Translational Mechanical Converter (TL) : fl_lib/Thermal Liquid/Elements/Translational Mechanical Converter (TL)  mech_orientation=1  interface_area=V/1000 m^2  x0=0 m  dead_volume=1e-5 m^3  environment_spec=1  environment_pressure=0.101325 MPa  dynamic_compressibility=1  T0=T0 C  p0=p0 bar
      settings: SourceProductName=Simscape  SourceProductBaseCode=SS
  Translational Damper : fl_lib/Mechanical/Translational Elements/Translational Damper  D=1e6 N/(m/s)  v_specify=off  v_priority=High  v=0 m/s  v_nominal_specify=off  v_nominal_unit=m/s  v_nominal_value=1  f_specify=off  f_priority=High  f=0 N  f_nominal_specify=off  f_nominal_unit=N  f_nominal_value=1
  Translational Hard Stop : fl_lib/Mechanical/Translational Elements/Translational Hard Stop  upper_bnd=1 m  lower_bnd=0 m  stiff_up=1e10 N/m  stiff_low=1e10 N/m  D_up=1500 N/(m/s)  D_low=1500 N/(m/s)  model=3  transition=0.1 mm  v_specify=off  v_priority=High  v=0 m/s  v_nominal_specify=off  v_nominal_unit=m/s  v_nominal_value=1  f_specify=off  f_priority=High  f=0 N  f_nominal_specify=off  f_nominal_unit=N  f_nominal_value=1  x_specify=on  x_priority=High  x=0 m  x_nominal_specify=off  x_nominal_unit=m  x_nominal_value=1
  Liquid : PMIOPort  Side=Left
  Out1 : Outport
  wires:
  Gain/1 -> Bus Creator/1  "Pression gaz [bar]"
  PS-Simulink Converter2/1 -> Bus Creator/3  "Position (0 à 1)"
  PS-Simulink Converter1/1 -> Bus Creator/2  "Température gaz"
  PS-Simulink Converter4/1 -> Gain/1
  Bus Creator/1 -> Out1/1
  Constant/1 -> Simulink-PS Converter3/1
  connections:
  PS-Simulink Converter2/LConn1 -- Ideal Translational Motion Sensor/RConn3
  PS-Simulink Converter1/LConn1 -- Pneumatic Pressure & Temperature Sensor/RConn3
  PS-Simulink Converter4/LConn1 -- Pneumatic Pressure & Temperature Sensor/RConn2
  Pneumatic Atmospheric Reference/LConn1 -- Pneumatic Pressure & Temperature Sensor/RConn1
  Ideal Temperature Source/LConn1 -- Pneumatic Piston Chamber/LConn3
  Pneumatic Pressure & Temperature Sensor/LConn1 -- Pneumatic Piston Chamber/LConn1 -- Gas Properties/RConn1
  Translational Hard Stop/LConn1 -- Translational Damper/RConn1 -- Pneumatic Piston Chamber/RConn1 -- Ideal Translational Motion Sensor/LConn1 -- Translational Mechanical Converter (TL)/RConn1 -- Mass/LConn1
  Translational Mechanical Converter (TL)/LConn2 -- Translational Damper/LConn1 -- Translational Hard Stop/RConn1 -- Mechanical Translational Reference/LConn1
  Translational Mechanical Converter (TL)/LConn1 -- Liquid/RConn1
  Translational Mechanical Converter (TL)/LConn3 -- Perfect Insulator/LConn1
  Ideal Translational Motion Sensor/RConn1 -- Pneumatic Piston Chamber/LConn2 -- Mechanical Translational Reference1/LConn1
  Thermal Reference/LConn1 -- Ideal Temperature Source/RConn2
  Simulink-PS Converter3/RConn1 -- Ideal Temperature Source/RConn1
  PS Terminator/LConn1 -- Ideal Translational Motion Sensor/RConn2

== system Library_SII_2018/Thermique/Capteur température ==
  Fcn : Fcn  Expr=u-273.16
  Ideal Temperature Sensor : fl_lib/Thermal/Thermal Sensors/Temperature Sensor
  PS-Simulink Converter : nesl_utility/PS-Simulink Converter  PhysicalDomain=network_engine_domain  SubClassName=ps_output  LeftPortType=input  RightPortType=output  PseudoPeriodic=off  Frequencies=[]  Unit=1  AffineConversion=off
  Thermal Reference : fl_lib/Thermal/Thermal Elements/Thermal Reference
  A : PMIOPort  Side=Left
  T [°C] : Outport
  wires:
  PS-Simulink Converter/1 -> Fcn/1
  Fcn/1 -> T [°C]/1
  connections:
  Ideal Temperature Sensor/RConn2 -- PS-Simulink Converter/LConn1
  Thermal Reference/LConn1 -- Ideal Temperature Sensor/RConn1
  A/RConn1 -- Ideal Temperature Sensor/LConn1

== system Library_SII_2018/Thermique/Incidence surface ==
  Energie soleil [W/m²] : Inport
  Hauteur soleil : Inport  Port=2
  Azimut soleil : Inport  Port=3
  orientation surface (nord = 0°) : Inport  Port=4
  inclinaison surface (horizontal = 0°) : Inport  Port=5
  Add : Sum  Inputs=+-
  Coefficient d'incidence : MATLAB Function  TreatAsAtomicUnit=on
  Display13 : Display
  Product : Product  RndMeth=Zero
  orientation : Constant  Value=180
  Energie surface [W/m²] : Outport
  wires:
  Coefficient d'incidence/1(CI) -> Product/1, Display13/1
  Product/1 -> Energie surface [W/m²]/1
  inclinaison surface (horizontal = 0°)/1 -> Coefficient d'incidence/1(i)
  orientation surface (nord = 0°)/1 -> Add/2
  orientation/1 -> Add/1
  Add/1 -> Coefficient d'incidence/2(o)
  Energie soleil [W/m²]/1 -> Product/2
  Hauteur soleil/1 -> Coefficient d'incidence/3(h)
  Azimut soleil/1 -> Coefficient d'incidence/4(a)

== system Library_SII_2018/Thermique/Paroi ==
  Add : Sum  Inputs=+-
  Conductive_ext : fl_lib/Thermal/Thermal Elements/Conductive Heat Transfer  area=s m^2  thickness=e/2 cm  th_cond=lambda W/(m*K)  T_specify=off  T_priority=High  T=0 K  T_nominal_specify=off  T_nominal_unit=K  T_nominal_value=1  Q_specify=off  Q_priority=High  Q=0 J/s  Q_nominal_specify=off  Q_nominal_unit=W  Q_nominal_value=1
      settings: SourceProductName=Simscape
  Conductive_int : fl_lib/Thermal/Thermal Elements/Conductive Heat Transfer  area=s m^2  thickness=e/2 cm  th_cond=lambda W/(m*K)  T_specify=off  T_priority=High  T=0 K  T_nominal_specify=off  T_nominal_unit=K  T_nominal_value=1  Q_specify=off  Q_priority=High  Q=0 J/s  Q_nominal_specify=off  Q_nominal_unit=W  Q_nominal_value=1
      settings: SourceProductName=Simscape
  Constant : Constant  Value=273.15
  Ideal Temperature Sensor : fl_lib/Thermal/Thermal Sensors/Temperature Sensor
  Inertie : fl_lib/Thermal/Thermal Elements/Thermal Mass  mass=masse kg  sp_heat=c J/kg/K  T_specify=on  T_priority=High  T=Ti degC  T_nominal_specify=off  T_nominal_unit=K  T_nominal_value=1  Q_specify=off  Q_priority=High  Q=0 J/s  Q_nominal_specify=off  Q_nominal_unit=W  Q_nominal_value=1
  PS-Simulink Converter : nesl_utility/PS-Simulink Converter  PhysicalDomain=network_engine_domain  SubClassName=ps_output  LeftPortType=input  RightPortType=output  PseudoPeriodic=off  Frequencies=[]  Unit=1  AffineConversion=on
  Thermal Reference1 : fl_lib/Thermal/Thermal Elements/Thermal Reference
  L : PMIOPort  Side=Left
  R : PMIOPort  Port=2  Side=Right
  T : Outport
  wires:
  Add/1 -> T/1
  Constant/1 -> Add/2
  PS-Simulink Converter/1 -> Add/1
  connections:
  Conductive_ext/LConn1 -- Conductive_int/RConn1 -- Inertie/LConn1 -- Ideal Temperature Sensor/LConn1
  L/RConn1 -- Conductive_int/LConn1
  R/RConn1 -- Conductive_ext/RConn1
  PS-Simulink Converter/LConn1 -- Ideal Temperature Sensor/RConn2
  Thermal Reference1/LConn1 -- Ideal Temperature Sensor/RConn1

== system Library_SII_2018/Thermique/Paroi (avec  rayonnement) ==
  Capacité : fl_lib/Thermal/Thermal Elements/Thermal Mass  mass=masse kg  sp_heat=c J/kg/K  T_specify=on  T_priority=High  T=Ti K  T_nominal_specify=off  T_nominal_unit=K  T_nominal_value=1  Q_specify=off  Q_priority=High  Q=0 J/s  Q_nominal_specify=off  Q_nominal_unit=W  Q_nominal_value=1
  Conduction ext : fl_lib/Thermal/Thermal Elements/Conductive Heat Transfer  area=s m^2  thickness=e/2 cm  th_cond=lambda W/(m*K)  T_specify=off  T_priority=High  T=0 K  T_nominal_specify=off  T_nominal_unit=K  T_nominal_value=1  Q_specify=off  Q_priority=High  Q=0 J/s  Q_nominal_specify=off  Q_nominal_unit=W  Q_nominal_value=1
      settings: SourceProductName=Simscape
  Conduction int : fl_lib/Thermal/Thermal Elements/Conductive Heat Transfer  area=s m^2  thickness=e/2 cm  th_cond=lambda W/(m*K)  T_specify=off  T_priority=High  T=0 K  T_nominal_specify=off  T_nominal_unit=K  T_nominal_value=1  Q_specify=off  Q_priority=High  Q=0 J/s  Q_nominal_specify=off  Q_nominal_unit=W  Q_nominal_value=1
      settings: SourceProductName=Simscape
  Ideal Heat Flow Sensor. : fl_lib/Thermal/Thermal Sensors/Heat Flow Rate Sensor
      settings: SourceProductName=Simscape  SourceProductBaseCode=SS
  Ideal Heat Flow Sensor.1 : fl_lib/Thermal/Thermal Sensors/Heat Flow Rate Sensor
      settings: SourceProductName=Simscape  SourceProductBaseCode=SS
  Ideal Temperature Sensor : fl_lib/Thermal/Thermal Sensors/Temperature Sensor
  PS-Simulink Converter : nesl_utility/PS-Simulink Converter  PhysicalDomain=network_engine_domain  SubClassName=ps_output  LeftPortType=input  RightPortType=output  PseudoPeriodic=off  Frequencies=[]  Unit=degC  AffineConversion=on
  PS2S : nesl_utility/PS-Simulink Converter  PhysicalDomain=network_engine_domain  SubClassName=ps_output  LeftPortType=input  RightPortType=output  PseudoPeriodic=off  Frequencies=[]  Unit=J/s  AffineConversion=off
  PS2S1 : nesl_utility/PS-Simulink Converter  PhysicalDomain=network_engine_domain  SubClassName=ps_output  LeftPortType=input  RightPortType=output  PseudoPeriodic=off  Frequencies=[]  Unit=J/s  AffineConversion=off
  Thermal Reference : fl_lib/Thermal/Thermal Elements/Thermal Reference
  Int : PMIOPort  Side=Left
  Ext : PMIOPort  Port=2  Side=Right
  Ray : PMIOPort  Port=3  Side=Right
  T : Outport
  Fext : Outport  Port=2
  Fint : Outport  Port=3
  wires:
  PS-Simulink Converter/1 -> T/1
  PS2S/1 -> Fext/1
  PS2S1/1 -> Fint/1
  connections:
  Thermal Reference/LConn1 -- Ideal Temperature Sensor/RConn1
  PS-Simulink Converter/LConn1 -- Ideal Temperature Sensor/RConn2
  Capacité/LConn1 -- Ideal Heat Flow Sensor.1/RConn2 -- Ray/RConn1 -- Ideal Temperature Sensor/LConn1 -- Ideal Heat Flow Sensor./LConn1
  Int/RConn1 -- Conduction int/LConn1
  Conduction ext/RConn1 -- Ext/RConn1
  Conduction ext/LConn1 -- Ideal Heat Flow Sensor./RConn2
  Ideal Heat Flow Sensor./RConn1 -- PS2S/LConn1
  Ideal Heat Flow Sensor.1/RConn1 -- PS2S1/LConn1
  Conduction int/RConn1 -- Ideal Heat Flow Sensor.1/LConn1
